simulink model "e6_taller_se"  (R2018a)
settings: Solver=VariableStepAuto  StartTime=0.0  StopTime=1  RelTol=1e-3
InitFcn:
  | ejercicio6_taller_se
values from neighbouring files (symbols this model uses):
  A = [-1/(R*C) -1/C;1/L 0]    [ejemplo_se.m]    (also in ejercicio6_taller_se.m = [-(1/C1)*(1/R1+1/R2) 1/(R2*C1); 1/(R2*C2) -1/(R2*C2)])
  B = [1/C 0]'    [ejemplo_se.m]    (also in ejercicio6_taller_se.m = [1/(R1*C1) 0]')
  C = 12e-6    (= 1.2e-05)    [ejemplo_se.m]    (also in ejercicio6_taller_se.m = [0 1])
  C1 = 10e-6    (= 1e-05)    [amp_op.m]    (also in ejercicio6_taller_se.m = 1e-06)
  C2 = 1e-6    (= 1e-06)    [amp_op.m]    (also in ejercicio6_taller_se.m = 1e-05)
  h = tf(-R3,[R1*R2*R3*C2*C1 C2*(R1*R3+R3*R2+R1*R2) R1])    [amp_op.m]    (also in ejemplo_se.m = tf(R,[R*C*L L R]); ejercicio6_taller_se.m = tf(1,[R1*R2*C1*C2 R1*(C1+C2)+R2*C2 1]))
  R1 = 100e3    (= 100000)    [amp_op.m]    (also in ejercicio6_taller_se.m = 10000)
  R2 = 1e3    (= 1000)    [amp_op.m]    (also in ejercicio6_taller_se.m = 5000)
settings Model: Creator=carma  LastModifiedBy=carma

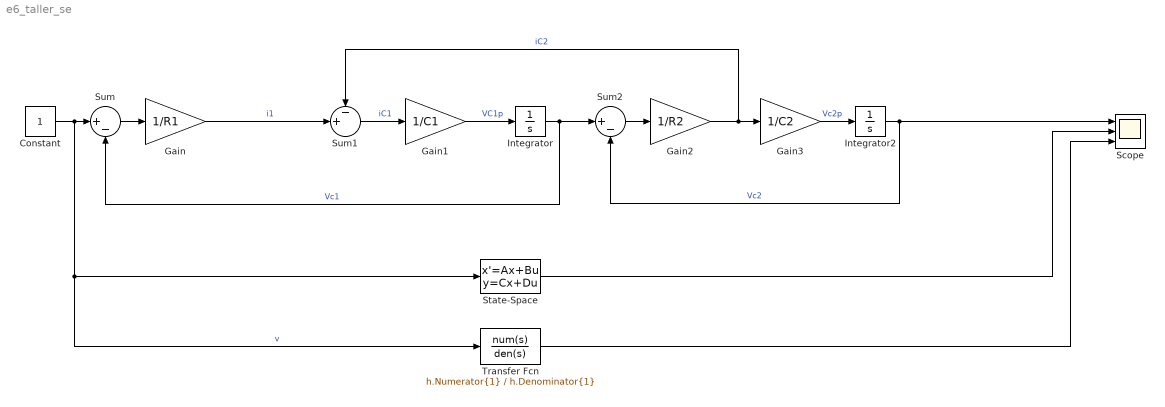
== system e6_taller_se ==
  Constant : Constant
  Gain : Gain  Gain=1/R1
  Gain1 : Gain  Gain=1/C1
  Gain2 : Gain  Gain=1/R2
  Gain3 : Gain  Gain=1/C2
  Integrator : Integrator
  Integrator2 : Integrator
  Scope : Scope  NumInputPorts=3
  State-Space : StateSpace  A=A  B=B  C=C  D=0  InitialCondition=0
  Sum : Sum  Inputs=|+-
  Sum1 : Sum  Inputs=-+|
  Sum2 : Sum  Inputs=|+-
  Transfer Fcn : TransferFcn  Numerator=h.Numerator{1}  Denominator=h.Denominator{1}
  wires:
  Sum/1 -> Gain/1
  Constant/1 -> Transfer Fcn/1, State-Space/1, Sum/1  "v"
  Integrator/1 -> Sum2/1, Sum/2  "Vc1"
  Gain/1 -> Sum1/2  "i1"
  Sum1/1 -> Gain1/1  "iC1"
  Gain1/1 -> Integrator/1  "VC1p"
  Gain2/1 -> Sum1/1, Gain3/1  "iC2"
  Sum2/1 -> Gain2/1
  Gain3/1 -> Integrator2/1  "Vc2p"
  Integrator2/1 -> Scope/1, Sum2/2  "Vc2"
  State-Space/1 -> Scope/2
  Transfer Fcn/1 -> Scope/3
